simulink model "verify_window_static_mdl"  (R2018b)
settings: Solver=ode45  StartTime=0  StopTime=24*3600  MaxStep=600  RelTol=1e-3  EnableMultiTasking=on
libraries: carnot x5
settings Model: Creator=drhf  LastModifiedBy=drhf
settings DataIOCC: LimitDataPoints=on  SaveFormat=Array
settings OptimizationCC: DefaultParameterBehavior=Inlined  LifeSpan=inf
settings DebuggingCC: UnderspecifiedInitializationDetection=Classic  MergeDetectMultiDrivingBlocksExec=none  SolverPrmCheckMsg=warning  SFUnexpectedBacktrackingDiag=warning  SFNoUnconditionalDefaultTransitionDiag=warning  SFExecutionAtInitializationDiag=none
settings HardwareCC: ProdBitPerPointer=32  ProdBitPerSizeT=32  ProdBitPerPtrDiffT=32  ProdLargestAtomicFloat=None  ProdIntDivRoundTo=Undefined  ProdEndianess=Unspecified  ProdWordSize=32  ProdHWDeviceType=32-bit Generic
settings ModelReferenceCC: PropagateSignalLabelsOutOfModel=off
settings SFSimCC: SimUseLocalCustomCode=off
settings RTWCC: RTWUseLocalCustomCode=off
settings CodeAppCC: StateflowObjectComments=on
settings GRTTargetCC: TargetLangStandard=C89/C90 (ANSI)  GeneratePreprocessorConditionals=Disable all
settings ConfigComp: CovMetricSettings=dw  CovHtmlReporting=on  CovSaveCumulativeToWorkspaceVar=on  CovSaveSingleToWorkspaceVar=on  CovExternalEMLEnable=off

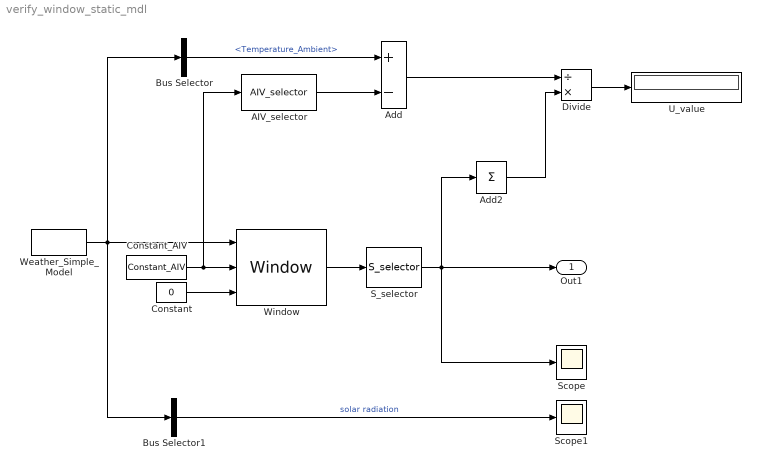
== system verify_window_static_mdl ==
  AIV_selector : carnot/Outputs/AIV_selector  e1=on  e2=off  e3=off  e4=off  e5=off  e6=off  e7=off  e8=off  e9=off
      settings: SourceProductName=Carnot
  Add : Sum  Inputs=+-
  Add2 : Sum  Inputs=1
  Bus Selector : BusSelector  OutputSignals=Temperature_Ambient
  Bus Selector1 : BusSelector  OutputSignals=Solar_Radiation_direct_surface,Solar_Radiation_diffuse_surface  OutputAsBus=on
  Constant : Constant  Value=0
  Constant_AIV : carnot/Source/Ventilation/Constant_AIV  Tsens=20  Tcon=20  Trad=20  mw=0.012  mco=0.01  rhoair=1.2  cpair=1004  pair=100000  nair=0.5
      settings: SourceProductName=Carnot
  Divide : Product  Inputs=/*
  S_selector : carnot/Outputs/S_selector  e1=off  e2=off  e3=off  e4=off  e5=off  e6=off  e7=on  e8=on  e9=off  e10=off  e11=off  e12=off  e13=off
      settings: SourceProductName=Carnot
  Scope : Scope
  Scope1 : Scope
  U_value : Display
  Weather_Simple_Model : carnot/Weather/Weather_Simple_Model  Ibn=900  Idg=100  tamb=0  deltaTsky=0  rh=50  precip="10e-3/24/3600           % 10 mm in 24 h"  cloud=0.125  p=1013e2  vw=5.85  wdir=270  lat=60  colangle=0  colazi=0  colrot=0
      settings: SourceProductName=Carnot
  Window : carnot/Basic/Thermal_Models/Window  pos=0  windowsize=[1 1]  frame=0.1  Ug=1.8  gvalue=0.6  tauzero=0.6*0.95  numpanes=2  d=[0.004 0.004]  rho=[2500 2500]  cp="[1008  1008]"  t0=20  misc=[0.2 0.1 1 1]  shad_type=No shading  type_glazing=double glazing normal  tau_shad=0.01  bli_a=0.05  bli_b=1  bli_c=0.05  bli_d=0.05  bli_alpha=90  bli_refl=0.2
      settings: SourceProductName=Carnot
  Out1 : Outport
  wires:
  Weather_Simple_Model/1 -> Window/1, Bus Selector/1, Bus Selector1/1
  Constant_AIV/1 -> Window/2, AIV_selector/1
  Window/1 -> S_selector/1
  S_selector/1 -> Out1/1, Scope/1, Add2/1
  AIV_selector/1 -> Add/2
  Add/1 -> Divide/1
  Add2/1 -> Divide/2
  Divide/1 -> U_value/1
  Constant/1 -> Window/3
  Bus Selector/1 -> Add/1  "<Temperature_Ambient>"
  Bus Selector1/1 -> Scope1/1  "solar radiation"
